simulink model "NSRwithPVC"  (R2018a)
settings: Solver=FixedStepDiscrete  StartTime=0.0  StopTime=10000  FixedStep=1  MaxStep=200.0  RelTol=1e-3
libraries: model_library x4
settings Model: Creator=Arsalan  LastModifiedBy=Arsalan

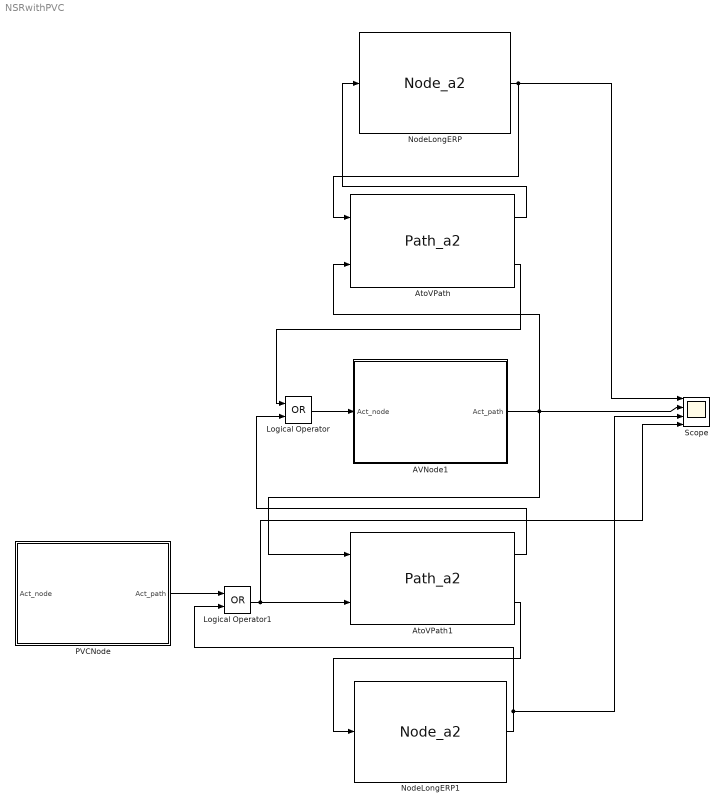
== system NSRwithPVC ==
  AVNode1 : Subsystem
  AtoVPath : model_library/Path_a2
      link override Tcond_def: Value=150
  AtoVPath1 : model_library/Path_a2
      link override Tcond_def: Value=150
  Logical Operator : Logic  Operator=OR  AllPortsSameDT=off  OutDataTypeStr=boolean
  Logical Operator1 : Logic  Operator=OR  AllPortsSameDT=off  OutDataTypeStr=boolean
  NodeLongERP : model_library/Node_a2
      link override ERP_def: Value=300
      link override Rest_def: Value=200
  NodeLongERP1 : model_library/Node_a2
      link override ERP_def: Value=300
      link override Rest_def: Value=2000
  PVCNode : Subsystem
  Scope : Scope  NumInputPorts=4
  wires:
  Logical Operator/1 -> AVNode1/1(Act_node)
  NodeLongERP/1 -> Scope/1, AtoVPath/1
  AtoVPath/1 -> NodeLongERP/1
  AtoVPath/2 -> Logical Operator/1
  AVNode1/1(Act_path) -> AtoVPath1/1, AtoVPath/2, Scope/2
  AtoVPath1/1 -> Logical Operator/2
  AtoVPath1/2 -> NodeLongERP1/1
  NodeLongERP1/1 -> Logical Operator1/2, Scope/3
  PVCNode/1(Act_path) -> Logical Operator1/1
  Logical Operator1/1 -> Scope/4, AtoVPath1/2

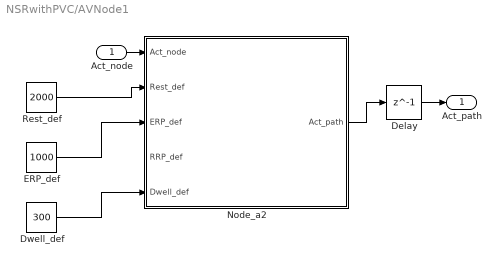
== system NSRwithPVC/AVNode1 ==
  Act_node : Inport
  Delay : Delay  DelayLength=1  InitialCondition=0
  Dwell_def : Constant  Value=300  OutDataTypeStr=uint16
  ERP_def : Constant  Value=1000  OutDataTypeStr=uint16
  Node_a2 : Stateflow chart  RequirementInfo={} %GIDa_edc28a8b_c2ed_4db7_b3ee_966bf724d5fb  TreatAsAtomicUnit=on
  Rest_def : Constant  Value=2000  OutDataTypeStr=uint16
  Act_path : Outport
  wires:
  Node_a2/1(Act_path) -> Delay/1
  Act_node/1 -> Node_a2/1(Act_node)
  Rest_def/1 -> Node_a2/2(Rest_def)
  ERP_def/1 -> Node_a2/3(ERP_def)
  Delay/1 -> Act_path/1
  Dwell_def/1 -> Node_a2/5(Dwell_def)

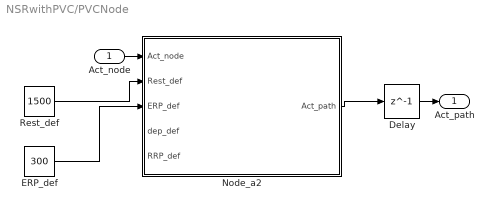
== system NSRwithPVC/PVCNode ==
  Act_node : Inport
  Delay : Delay  DelayLength=1  InitialCondition=0
  ERP_def : Constant  Value=300  OutDataTypeStr=uint16
  Node_a2 : Stateflow chart  RequirementInfo="{}  %GIDa_6ee29377_7781_44c0_ad76_b00d26592997"  TreatAsAtomicUnit=on
  Rest_def : Constant  Value=1500  OutDataTypeStr=uint16
  Act_path : Outport
  wires:
  Node_a2/1(Act_path) -> Delay/1
  Act_node/1 -> Node_a2/1(Act_node)
  Rest_def/1 -> Node_a2/2(Rest_def)
  ERP_def/1 -> Node_a2/3(ERP_def)
  Delay/1 -> Act_path/1

== stateflow chart NSRwithPVC/AVNode1/Node_a2 ==
  state node
    settings: description=|
        | temp can be thought of a sub-mode of ERP, which only exists to make sure that act_path is high for one period.
        | 
        | In ERP, if Act_node is received, then it is ignored through that self-transition.
        | 
        | Note this doesn't model variations in cycle length because everytime it is stimulated in RRP, ERP_cur is set to ERP_def again.
    state Rest
    state Dwell
    state RRP
    state ERP
    state temp
    (default) -> Rest : {Rest_cur=Rest_def; Dwell_cur=Dwell_def;}
    Dwell -> Dwell [order 2] : [Dwell_cur>uint16(0)]/{Dwell_cur=Dwell_cur-uint16(1);}
    Rest -> Dwell [order 3] : [Act_node==false && Rest_cur<=uint16(0)]
    Rest -> Dwell [order 1] : [Act_node==true]
    Rest -> Rest [order 2] : [Act_node==false && Rest_cur>uint16(0)]/{Rest_cur = Rest_cur - uint16(1);}
    RRP -> Dwell [order 3] : [Act_node==true]
    RRP -> Rest [order 1] : [RRP_cur<=0]/{Rest_cur=Rest_def;}
    Dwell -> temp [order 1] : [Dwell_cur<=uint16(0)]/{Act_path=true;uptime= uint16(0);Dwell_cur=Dwell_def;uptime= uint16(0);ERP_cur=ERP_def;}
    RRP -> RRP [order 2] : [Act_node==false && RRP_cur>0]/{RRP_cur=RRP_cur-uint16(1);}
    ERP -> RRP [order 1] : [ERP_cur<=uint16(0)]/{RRP_cur=RRP_def;}
    temp -> temp [order 1] : [uptime<uint16(1)]/{uptime = uptime + uint16(1);ERP_cur =ERP_cur - uint16(1);}
    temp -> ERP [order 2] : [uptime>=uint16(1)]/{Act_path=false;}
    ERP -> ERP [order 3] : [Act_node==true]
    ERP -> ERP [order 2] : {ERP_cur = ERP_cur - uint16(1);}
  data: Act_node input boolean; Act_path output boolean; Rest_cur local uint16; ERP_cur local uint16; Rest_def input uint16; ERP_def input uint16; uptime local uint16; RRP_cur local uint16; RRP_def input uint16; Dwell_cur local uint16; Dwell_def input uint16

== stateflow chart NSRwithPVC/PVCNode/Node_a2 ==
  state node
    settings: description=|
        | temp can be thought of a sub-mode of ERP, which only exists to make sure that act_path is high for one period.
        | 
        | In ERP, if Act_node is received, then it is ignored through that self-transition.
        | 
        | Note this doesn't model variations in cycle length because everytime it is stimulated in RRP, ERP_cur is set to ERP_def again.
    state Rest
    state RRP
    state ERP
    state temp
    (default) -> Rest : {Rest_cur=Rest_def;}
    Rest -> temp [order 3] : [Act_node==false && Rest_cur<=uint16(0)]/{Act_path=true;uptime= uint16(0);ERP_cur=ERP_def;}
    Rest -> temp [order 1] : [Act_node==true]/{Act_path=true;uptime= uint16(0);ERP_cur=ERP_def;}
    Rest -> Rest [order 2] : [Act_node==false && Rest_cur>uint16(0)]/{Rest_cur = Rest_cur - uint16(1);}
    RRP -> Rest [order 1] : [RRP_cur<=0]/{Rest_cur=Rest_def;}
    RRP -> RRP [order 2] : [Act_node==false && RRP_cur>0]/{RRP_cur=RRP_cur-uint16(1);}
    RRP -> temp [order 3] : [Act_node==true]/{Act_path=true;uptime= uint16(0);ERP_cur=ERP_def;}
    ERP -> RRP [order 1] : [ERP_cur<=uint16(0)]/{RRP_cur=RRP_def;}
    temp -> temp [order 1] : [uptime<uint16(1)]/{uptime = uptime + uint16(1);ERP_cur =ERP_cur - uint16(1);}
    temp -> ERP [order 2] : [uptime>=uint16(1)]/{Act_path=false;}
    ERP -> ERP [order 3] : [Act_node==true]
    ERP -> ERP [order 2] : {ERP_cur = ERP_cur - uint16(1);}
  data: Act_node input boolean; Act_path output boolean; Rest_cur local uint16; ERP_cur local uint16; Rest_def input uint16; ERP_def input uint16; uptime local uint16; dep_cur local uint16; dep_def input uint16; RRP_cur local uint16; RRP_def input uint16
